simulink model "QRT_sim_test1"  (Simulink 10.3)
settings: Solver=ode45  StartTime=0.0  StopTime=10  RelTol=1e-3  EnableMultiTasking=on
libraries: pid_lib x4
settings Model: Creator=page365  LastModifiedBy=helle
settings DataIOCC: LimitDataPoints=on
settings DebuggingCC: SolverPrmCheckMsg=warning
settings SFSimCC: SimParseCustomCode=off

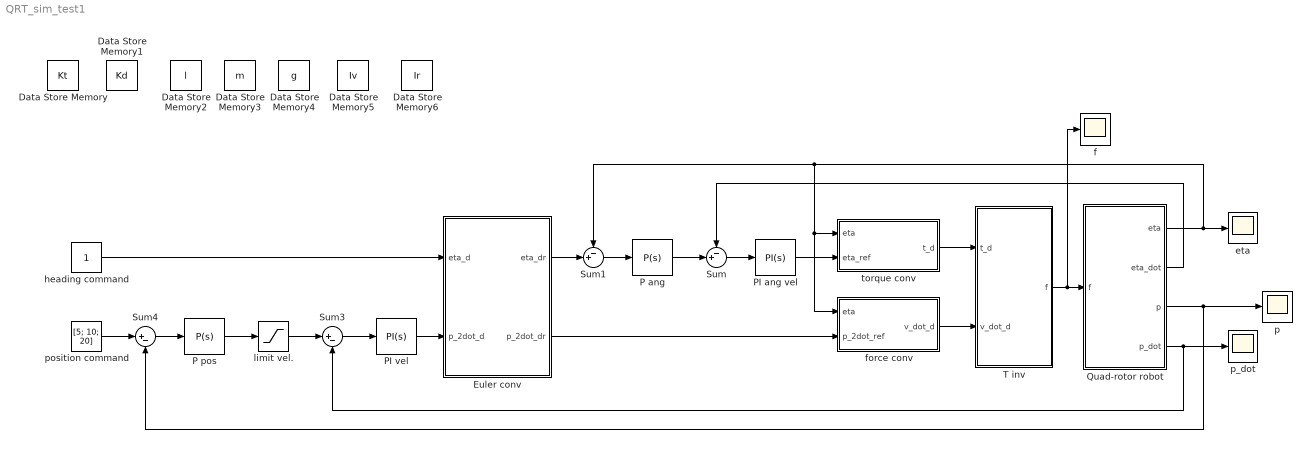
== system QRT_sim_test1 ==
  Data Store Memory : DataStoreMemory  DataStoreName=Kt  InitialValue=1  ShowAdditionalParam=off  OutDataTypeStr=double
  Data Store Memory1 : DataStoreMemory  DataStoreName=Kd  InitialValue=0.2  ShowAdditionalParam=off  OutDataTypeStr=double
  Data Store Memory2 : DataStoreMemory  DataStoreName=l  InitialValue=0.3  ShowAdditionalParam=off  OutDataTypeStr=double
  Data Store Memory3 : DataStoreMemory  DataStoreName=m  InitialValue=2.2  ShowAdditionalParam=off  OutDataTypeStr=double
  Data Store Memory4 : DataStoreMemory  DataStoreName=g  InitialValue=[0; 0; -9.81]  ShowAdditionalParam=off  OutDataTypeStr=double
  Data Store Memory5 : DataStoreMemory  DataStoreName=Iv  InitialValue=[0.0170 0 0; 0 0.0170 0; 0 0 0.0230]  ShowAdditionalParam=off  OutDataTypeStr=double
  Data Store Memory6 : DataStoreMemory  DataStoreName=Ir  InitialValue=[0.001 0 0; 0 0.001 0; 0 0 0.001]  ShowAdditionalParam=off  OutDataTypeStr=double
  Euler conv : MATLAB Function  TreatAsAtomicUnit=on
  P ang : pid_lib/PID Controller  Controller=P  Form=Parallel  TimeDomain=Continuous-time  UseExternalTs=off  SampleTime=1  IntegratorMethod=Forward Euler  FilterMethod=Forward Euler  ControllerParametersSource=internal  P=5  I=0.00102076543610064  D=0  UseFilter=on  N=100  TunerSelectOption=Transfer Function Based (PID Tuner App)  InitialConditionSource=internal  InitialConditionForIntegrator=0  InitialConditionForFilter=0  DifferentiatorICPrevScaledInput=0  ExternalReset=none  TrackingMode=off  Kt=1  LimitOutput=off  SatLimitsSource=internal  UpperSaturationLimit=inf  LowerSaturationLimit=-inf  LinearizeAsGain=off  AntiWindupMode=none  Kb=1  POutMin=[]  POutMax=[]  IOutMin=[]  IOutMax=[]  DOutMin=[]  DOutMax=[]  NOutMin=[]  NOutMax=[]  SumOutMin=[]  SumOutMax=[]  SaturationOutMin=[]  SaturationOutMax=[]  PParamMin=[]  PParamMax=[]  IParamMin=[]  IParamMax=[]  DParamMin=[]  DParamMax=[]  NParamMin=[]  NParamMax=[]  KbParamMin=[]  KbParamMax=[]  KtParamMin=[]  KtParamMax=[]  KbOutMin=[]  KbOutMax=[]  KtOutMin=[]  KtOutMax=[]  IntegratorOutMin=[]  IntegratorOutMax=[]  FilterOutMin=[]  FilterOutMax=[]  SumI1OutMin=[]  SumI1OutMax=[]  SumI2OutMin=[]  SumI2OutMax=[]  SumI3OutMin=[]  SumI3OutMax=[]  SumI4OutMin=[]  SumI4OutMax=[]  SumDOutMin=[]  SumDOutMax=[]  DifferentiatorOutMin=[]  DifferentiatorOutMax=[]  FilterDiffOutCoefMin=[]  FilterDiffOutCoefMax=[]  ReciprocalOutMin=[]  ReciprocalOutMax=[]  SumDenOutMin=[]  SumDenOutMax=[]  SumNumOutMin=[]  SumNumOutMax=[]  DivideOutMin=[]  DivideOutMax=[]  UdiffTsProdOutMin=[]  UdiffTsProdOutMax=[]  NTsProdOutMin=[]  NTsProdOutMax=[]  UintegralTsProdOutMin=[]  UintegralTsProdOutMax=[]  UngainTsProdOutMin=[]  UngainTsProdOutMax=[]  IntegratorContinuousStateAttributes=''  IntegratorStateMustResolveToSignalObject=off  IntegratorRTWStateStorageClass=Auto  FilterContinuousStateAttributes=''  FilterStateMustResolveToSignalObject=off  FilterRTWStateStorageClass=Auto  ParallelPVariant=InternalParameters  IdealPVariant=Disabled  IVariant=Disabled  DVariant=Disabled  IntegratorVariant=Disabled  SatVariant=Disabled  AWVariant=Disabled  PCopyVariant=Disabled  TRVariant=Disabled  FdbkBlocksVariant=Forward  IdealPFdbkVariant=Disabled  SatFdbkVariant=Disabled  DerivativeFilterVariant=Disabled  NVariant=Disabled  NCopyVariant=Disabled_SignalSpec  FilterICVariant=Disabled  IntegratorICVariant=Disabled  ExternalResetVariant=Disabled  TRSumVariant=Passthrough  SumFdbkVariant=Disabled  SumVariant=Passthrough_P  TsampFilterVariant=InternalTs  TsampNgainVariant=Passthrough  TsampIntegralVariant=Disabled_SignalSpec  ExternalSaturationOutDataTypeStr=Inherit: Same as second input
  P pos : pid_lib/PID Controller  Controller=P  Form=Parallel  TimeDomain=Continuous-time  UseExternalTs=off  SampleTime=1  IntegratorMethod=Forward Euler  FilterMethod=Forward Euler  ControllerParametersSource=internal  P=1  I=0.00102076543610064  D=0  UseFilter=on  N=100  TunerSelectOption=Transfer Function Based (PID Tuner App)  InitialConditionSource=internal  InitialConditionForIntegrator=0  InitialConditionForFilter=0  DifferentiatorICPrevScaledInput=0  ExternalReset=none  TrackingMode=off  Kt=1  LimitOutput=off  SatLimitsSource=internal  UpperSaturationLimit=inf  LowerSaturationLimit=-inf  LinearizeAsGain=off  AntiWindupMode=none  Kb=1  POutMin=[]  POutMax=[]  IOutMin=[]  IOutMax=[]  DOutMin=[]  DOutMax=[]  NOutMin=[]  NOutMax=[]  SumOutMin=[]  SumOutMax=[]  SaturationOutMin=[]  SaturationOutMax=[]  PParamMin=[]  PParamMax=[]  IParamMin=[]  IParamMax=[]  DParamMin=[]  DParamMax=[]  NParamMin=[]  NParamMax=[]  KbParamMin=[]  KbParamMax=[]  KtParamMin=[]  KtParamMax=[]  KbOutMin=[]  KbOutMax=[]  KtOutMin=[]  KtOutMax=[]  IntegratorOutMin=[]  IntegratorOutMax=[]  FilterOutMin=[]  FilterOutMax=[]  SumI1OutMin=[]  SumI1OutMax=[]  SumI2OutMin=[]  SumI2OutMax=[]  SumI3OutMin=[]  SumI3OutMax=[]  SumI4OutMin=[]  SumI4OutMax=[]  SumDOutMin=[]  SumDOutMax=[]  DifferentiatorOutMin=[]  DifferentiatorOutMax=[]  FilterDiffOutCoefMin=[]  FilterDiffOutCoefMax=[]  ReciprocalOutMin=[]  ReciprocalOutMax=[]  SumDenOutMin=[]  SumDenOutMax=[]  SumNumOutMin=[]  SumNumOutMax=[]  DivideOutMin=[]  DivideOutMax=[]  UdiffTsProdOutMin=[]  UdiffTsProdOutMax=[]  NTsProdOutMin=[]  NTsProdOutMax=[]  UintegralTsProdOutMin=[]  UintegralTsProdOutMax=[]  UngainTsProdOutMin=[]  UngainTsProdOutMax=[]  IntegratorContinuousStateAttributes=''  IntegratorStateMustResolveToSignalObject=off  IntegratorRTWStateStorageClass=Auto  FilterContinuousStateAttributes=''  FilterStateMustResolveToSignalObject=off  FilterRTWStateStorageClass=Auto  ParallelPVariant=InternalParameters  IdealPVariant=Disabled  IVariant=Disabled  DVariant=Disabled  IntegratorVariant=Disabled  SatVariant=Disabled  AWVariant=Disabled  PCopyVariant=Disabled  TRVariant=Disabled  FdbkBlocksVariant=Forward  IdealPFdbkVariant=Disabled  SatFdbkVariant=Disabled  DerivativeFilterVariant=Disabled  NVariant=Disabled  NCopyVariant=Disabled_SignalSpec  FilterICVariant=Disabled  IntegratorICVariant=Disabled  ExternalResetVariant=Disabled  TRSumVariant=Passthrough  SumFdbkVariant=Disabled  SumVariant=Passthrough_P  TsampFilterVariant=InternalTs  TsampNgainVariant=Passthrough  TsampIntegralVariant=Disabled_SignalSpec  ExternalSaturationOutDataTypeStr=Inherit: Same as second input
  PI ang vel : pid_lib/PID Controller  Controller=PI  Form=Parallel  TimeDomain=Continuous-time  UseExternalTs=off  SampleTime=1  IntegratorMethod=Forward Euler  FilterMethod=Forward Euler  ControllerParametersSource=internal  P=20  I=100  D=0  UseFilter=on  N=100  TunerSelectOption=Transfer Function Based (PID Tuner App)  InitialConditionSource=internal  InitialConditionForIntegrator=0  InitialConditionForFilter=0  DifferentiatorICPrevScaledInput=0  ExternalReset=none  TrackingMode=off  Kt=1  LimitOutput=off  SatLimitsSource=internal  UpperSaturationLimit=inf  LowerSaturationLimit=-inf  LinearizeAsGain=off  AntiWindupMode=none  Kb=1  POutMin=[]  POutMax=[]  IOutMin=[]  IOutMax=[]  DOutMin=[]  DOutMax=[]  NOutMin=[]  NOutMax=[]  SumOutMin=[]  SumOutMax=[]  SaturationOutMin=[]  SaturationOutMax=[]  PParamMin=[]  PParamMax=[]  IParamMin=[]  IParamMax=[]  DParamMin=[]  DParamMax=[]  NParamMin=[]  NParamMax=[]  KbParamMin=[]  KbParamMax=[]  KtParamMin=[]  KtParamMax=[]  KbOutMin=[]  KbOutMax=[]  KtOutMin=[]  KtOutMax=[]  IntegratorOutMin=[]  IntegratorOutMax=[]  FilterOutMin=[]  FilterOutMax=[]  SumI1OutMin=[]  SumI1OutMax=[]  SumI2OutMin=[]  SumI2OutMax=[]  SumI3OutMin=[]  SumI3OutMax=[]  SumI4OutMin=[]  SumI4OutMax=[]  SumDOutMin=[]  SumDOutMax=[]  DifferentiatorOutMin=[]  DifferentiatorOutMax=[]  FilterDiffOutCoefMin=[]  FilterDiffOutCoefMax=[]  ReciprocalOutMin=[]  ReciprocalOutMax=[]  SumDenOutMin=[]  SumDenOutMax=[]  SumNumOutMin=[]  SumNumOutMax=[]  DivideOutMin=[]  DivideOutMax=[]  UdiffTsProdOutMin=[]  UdiffTsProdOutMax=[]  NTsProdOutMin=[]  NTsProdOutMax=[]  UintegralTsProdOutMin=[]  UintegralTsProdOutMax=[]  UngainTsProdOutMin=[]  UngainTsProdOutMax=[]  IntegratorContinuousStateAttributes=''  IntegratorStateMustResolveToSignalObject=off  IntegratorRTWStateStorageClass=Auto  FilterContinuousStateAttributes=''  FilterStateMustResolveToSignalObject=off  FilterRTWStateStorageClass=Auto  ParallelPVariant=InternalParameters  IdealPVariant=Disabled  IVariant=InternalParameters  DVariant=Disabled  IntegratorVariant=Continuous  SatVariant=Disabled  AWVariant=Passthrough  PCopyVariant=Disabled  TRVariant=Disabled  FdbkBlocksVariant=Forward  IdealPFdbkVariant=Disabled  SatFdbkVariant=Disabled  DerivativeFilterVariant=Disabled  NVariant=Disabled  NCopyVariant=Disabled_SignalSpec  FilterICVariant=Disabled  IntegratorICVariant=InternalICs  ExternalResetVariant=Disabled  TRSumVariant=Passthrough  SumFdbkVariant=Disabled  SumVariant=Sum_PI  TsampFilterVariant=InternalTs  TsampNgainVariant=Passthrough  TsampIntegralVariant=Passthrough  ExternalSaturationOutDataTypeStr=Inherit: Same as second input
  PI vel : pid_lib/PID Controller  Controller=PI  Form=Parallel  TimeDomain=Continuous-time  UseExternalTs=off  SampleTime=1  IntegratorMethod=Forward Euler  FilterMethod=Forward Euler  ControllerParametersSource=internal  P=2  I=0  D=0  UseFilter=on  N=100  TunerSelectOption=Transfer Function Based (PID Tuner App)  InitialConditionSource=internal  InitialConditionForIntegrator=0  InitialConditionForFilter=0  DifferentiatorICPrevScaledInput=0  ExternalReset=none  TrackingMode=off  Kt=1  LimitOutput=off  SatLimitsSource=internal  UpperSaturationLimit=inf  LowerSaturationLimit=-inf  LinearizeAsGain=off  AntiWindupMode=none  Kb=1  POutMin=[]  POutMax=[]  IOutMin=[]  IOutMax=[]  DOutMin=[]  DOutMax=[]  NOutMin=[]  NOutMax=[]  SumOutMin=[]  SumOutMax=[]  SaturationOutMin=[]  SaturationOutMax=[]  PParamMin=[]  PParamMax=[]  IParamMin=[]  IParamMax=[]  DParamMin=[]  DParamMax=[]  NParamMin=[]  NParamMax=[]  KbParamMin=[]  KbParamMax=[]  KtParamMin=[]  KtParamMax=[]  KbOutMin=[]  KbOutMax=[]  KtOutMin=[]  KtOutMax=[]  IntegratorOutMin=[]  IntegratorOutMax=[]  FilterOutMin=[]  FilterOutMax=[]  SumI1OutMin=[]  SumI1OutMax=[]  SumI2OutMin=[]  SumI2OutMax=[]  SumI3OutMin=[]  SumI3OutMax=[]  SumI4OutMin=[]  SumI4OutMax=[]  SumDOutMin=[]  SumDOutMax=[]  DifferentiatorOutMin=[]  DifferentiatorOutMax=[]  FilterDiffOutCoefMin=[]  FilterDiffOutCoefMax=[]  ReciprocalOutMin=[]  ReciprocalOutMax=[]  SumDenOutMin=[]  SumDenOutMax=[]  SumNumOutMin=[]  SumNumOutMax=[]  DivideOutMin=[]  DivideOutMax=[]  UdiffTsProdOutMin=[]  UdiffTsProdOutMax=[]  NTsProdOutMin=[]  NTsProdOutMax=[]  UintegralTsProdOutMin=[]  UintegralTsProdOutMax=[]  UngainTsProdOutMin=[]  UngainTsProdOutMax=[]  IntegratorContinuousStateAttributes=''  IntegratorStateMustResolveToSignalObject=off  IntegratorRTWStateStorageClass=Auto  FilterContinuousStateAttributes=''  FilterStateMustResolveToSignalObject=off  FilterRTWStateStorageClass=Auto  ParallelPVariant=InternalParameters  IdealPVariant=Disabled  IVariant=InternalParameters  DVariant=Disabled  IntegratorVariant=Continuous  SatVariant=Disabled  AWVariant=Passthrough  PCopyVariant=Disabled  TRVariant=Disabled  FdbkBlocksVariant=Forward  IdealPFdbkVariant=Disabled  SatFdbkVariant=Disabled  DerivativeFilterVariant=Disabled  NVariant=Disabled  NCopyVariant=Disabled_SignalSpec  FilterICVariant=Disabled  IntegratorICVariant=InternalICs  ExternalResetVariant=Disabled  TRSumVariant=Passthrough  SumFdbkVariant=Disabled  SumVariant=Sum_PI  TsampFilterVariant=InternalTs  TsampNgainVariant=Passthrough  TsampIntegralVariant=Passthrough  ExternalSaturationOutDataTypeStr=Inherit: Same as second input
  Quad-rotor robot : Subsystem
  Sum : Sum  Inputs=-+|
  Sum1 : Sum  Inputs=-+|
  Sum3 : Sum  Inputs=|+-
  Sum4 : Sum  Inputs=|+-
  T inv : MATLAB Function  TreatAsAtomicUnit=on
  eta : Scope
  f : Scope
  force conv : MATLAB Function  TreatAsAtomicUnit=on
  heading command : Constant
  limit vel. : Saturate  UpperLimit=5  LowerLimit=-5
  p : Scope
  p_dot : Scope
  position command : Constant  Value=[5; 10; 20]
  torque conv : MATLAB Function  TreatAsAtomicUnit=on
  wires:
  T inv/1(f) -> f/1, Quad-rotor robot/1(f)
  torque conv/1(t_d) -> T inv/1(t_d)
  force conv/1(v_dot_d) -> T inv/2(v_dot_d)
  Quad-rotor robot/2(eta_dot) -> Sum/1
  Quad-rotor robot/1(eta) -> force conv/1(eta), torque conv/1(eta), Sum1/1, eta/1
  Sum1/1 -> P ang/1
  Quad-rotor robot/4(p_dot) -> p_dot/1, Sum3/2
  PI ang vel/1 -> torque conv/2(eta_ref)
  Sum/1 -> PI ang vel/1
  P ang/1 -> Sum/2
  Euler conv/1(eta_dr) -> Sum1/2
  Sum4/1 -> P pos/1
  Sum3/1 -> PI vel/1
  position command/1 -> Sum4/1
  Euler conv/2(p_2dot_dr) -> force conv/2(p_2dot_ref)
  PI vel/1 -> Euler conv/2(p_2dot_d)
  heading command/1 -> Euler conv/1(eta_d)
  P pos/1 -> limit vel./1
  Quad-rotor robot/3(p) -> p/1, Sum4/2
  limit vel./1 -> Sum3/1

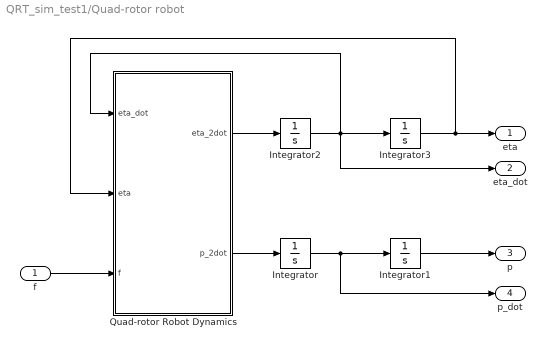
== system QRT_sim_test1/Quad-rotor robot ==
  f : Inport
  Integrator{,1..3} (4 alike) : Integrator
  Quad-rotor Robot Dynamics : MATLAB Function  TreatAsAtomicUnit=on
  eta : Outport
  eta_dot : Outport  Port=2
  p : Outport  Port=3
  p_dot : Outport  Port=4
  wires:
  Integrator/1 -> Integrator1/1, p_dot/1
  Integrator1/1 -> p/1
  Quad-rotor Robot Dynamics/2(p_2dot) -> Integrator/1
  Quad-rotor Robot Dynamics/1(eta_2dot) -> Integrator2/1
  Integrator2/1 -> Integrator3/1, eta_dot/1, Quad-rotor Robot Dynamics/1(eta_dot)
  Integrator3/1 -> eta/1, Quad-rotor Robot Dynamics/2(eta)
  f/1 -> Quad-rotor Robot Dynamics/3(f)

== matlab function T inv ==
  settings: updateMethod=DISCRETE
  data: t_d input double size=3; f output double size=4; v_dot_d input double size=1; Kd data_store_memory double size=1; l data_store_memory double size=1; m data_store_memory double size=1
function f = fcn(t_d, v_dot_d)

global Kd l m

r = Kd;

T = [1/m  1/m  1/m  1/m;
     0    -l   0    l;
     -l   0    l    0;
     r    -r   r    -r];

u = [v_dot_d(1,1); t_d(1,1); t_d(2,1); t_d(3,1)]; 
 
f = inv(T)*u;

% limits min and max force from rotor
% because motor can't make unlimited force
min_f = 0;
max_f = 10;

if (f(1,1) < min_f) f(1,1) = min_f; end
if (f(2,1) < min_f) f(2,1) = min_f; end
if (f(3,1) < min_f) f(3,1) = min_f; end
if (f(4,1) < min_f) f(4,1) = min_f; end

if (f(1,1) > max_f) f(1,1) = max_f; end
if (f(2,1) > max_f) f(2,1) = max_f; end
if (f(3,1) > max_f) f(3,1) = max_f; end
if (f(4,1) > max_f) f(4,1) = max_f; end

== matlab function Quad-rotor robot/Quad-rotor Robot Dynamics ==
  settings: updateMethod=DISCRETE
  data: eta_dot input double size=3; eta_2dot output double size=3; eta input double size=3; p_2dot output double size=3; f input double size=4; Kt data_store_memory double; Kd data_store_memory double; l data_store_memory double; m data_store_memory double; g data_store_memory double; Iv data_store_memory double; Ir data_store_memory double
function [eta_2dot, p_2dot] = fcn(eta_dot, eta, f)

global Kt Kd l m g Iv Ir;
  
phi_dot = eta_dot(1,1);
theta_dot = eta_dot(2,1);
psi_dot = eta_dot(3,1);

sphi = sin(eta(1,1));
cphi = cos(eta(1,1));
stht = sin(eta(2,1));
ctht = cos(eta(2,1));
spsi = sin(eta(3,1));
cpsi = cos(eta(3,1));

R = [cpsi*ctht cpsi*stht*sphi-spsi*cphi cpsi*stht*cphi+spsi*sphi;	
     spsi*ctht spsi*stht*sphi+cpsi*cphi spsi*stht*cphi-cpsi*sphi;	
     -stht     ctht*sphi                ctht*cphi];

C = [1 0     -stht;
     0 cphi  sphi*ctht;
     0 -sphi cphi*ctht];
 
C_dot = [0 0             -theta_dot*ctht;
         0 -phi_dot*sphi phi_dot*cphi*ctht-theta_dot*sphi*stht;
         0 -phi_dot*cphi -phi_dot*sphi*ctht-theta_dot*cphi*stht];

F1 = Kt*f(1,1);
F2 = Kt*f(2,1);
F3 = Kt*f(3,1);
F4 = Kt*f(4,1);
     
t1 = Kd*f(1,1);
t2 = Kd*f(2,1);
t3 = Kd*f(3,1);
t4 = Kd*f(4,1);
     
F = [0; 0; F1+F2+F3+F4];
Q = [l*(F4-F2); l*(F3-F1); t1-t2+t3-t4];
 
p_2dot = g + R*F/m;
eta_2dot = inv(Iv*C)*Q;

== matlab function torque conv ==
  settings: updateMethod=DISCRETE
  data: eta input double size=3; eta_ref input double size=3; t_d output double size=3; Iv data_store_memory double size=3
function t_d = fcn(eta, eta_ref)

global Iv;

sphi = sin(eta(1,1));
cphi = cos(eta(1,1));
stht = sin(eta(2,1));
ctht = cos(eta(2,1));
spsi = sin(eta(3,1));
cpsi = cos(eta(3,1));

C = [1   0     -stht;
     0   cphi  sphi*ctht;
     0   -sphi cphi*ctht];

t_d = Iv*C*eta_ref;

== matlab function force conv ==
  data: eta input double size=3; p_2dot_ref input double size=1; v_dot_d output double size=1
function v_dot_d = fcn(eta, p_2dot_ref)

sphi = sin(eta(1,1));
cphi = cos(eta(1,1));
stht = sin(eta(2,1));
ctht = cos(eta(2,1));
spsi = sin(eta(3,1));
cpsi = cos(eta(3,1));

R = [cpsi*ctht cpsi*stht*sphi-spsi*cphi cpsi*stht*cphi+spsi*sphi;	
     spsi*ctht spsi*stht*sphi+cpsi*cphi spsi*stht*cphi-cpsi*sphi;	
     -stht     ctht*sphi                ctht*cphi];

u = [0; 0; p_2dot_ref(1,1)];
d = R'*u;

v_dot_d = d(3,1);

== matlab function Euler conv ==
  data: eta_d input double size=1; p_2dot_d input double size=3; eta_dr output double size=3; p_2dot_dr output double size=1
function [eta_dr, p_2dot_dr] = fcn(eta_d, p_2dot_d)
%#eml

psi_d = eta_d(1,1);

x_2dot_d = p_2dot_d(1,1);
y_2dot_d = p_2dot_d(2,1);
z_2dot_d = p_2dot_d(3,1) + 9.81;

d = sqrt(x_2dot_d*x_2dot_d + y_2dot_d*y_2dot_d + z_2dot_d*z_2dot_d);

if (-0.001 < d & d < 0.001)
    phi_d_ref = 0;
else
    phi_d_ref = asin((x_2dot_d*sin(psi_d) - y_2dot_d*cos(psi_d))/d);
end

theta_dr = atan2(x_2dot_d*cos(psi_d) + y_2dot_d*sin(psi_d), z_2dot_d);

min_ang = -pi/6;
max_ang =  pi/6;

if (phi_d_ref < min_ang) phi_d_ref = min_ang; end
if (phi_d_ref > max_ang) phi_d_ref = max_ang; end

if (theta_dr < min_ang) theta_dr = min_ang; end
if (theta_dr > max_ang) theta_dr = max_ang; end

eta_dr   = [phi_d_ref; theta_dr; psi_d];
p_2dot_dr = [z_2dot_d];
